simulink model "e5_Quadrotor_stable_nn_cex"  (R2020a)
settings: Solver=FixedStepAuto  StartTime=0.0  StopTime=options.T_train  FixedStep=options.dt  RelTol=1e-6
undefined symbols (not defined in the file or in its folder): options, Quad
libraries: neural x179, simulink x3
(part 5 of 10)

== system e5_Quadrotor_stable_nn_cex/NN/Layer 2/Delays 1 ==
  "p{2}" : Inport  PortDimensions=50
      mask Display: e = 0.06;c1 = [120 230 180]/255;c2 = ([120 230 180]+0)/(256+128);c3 = ([120 230 180]+128)/(256+128);patch([0 1 1 0],[0 0 1 1],c1);patch([0 1 1 1-e 1-e 0+e],[0 0 1 1-e 0+e 0+e],c2);patch([0 0 1 1-e 0+e 0+e],[0 1 1 1-e 1-e 0+e],c3);plot([0 1 1 0 0],[0 0 1 1 0]);
  mux : Mux  Inputs=1
      mask Display: e = 0.06;c1 = [120 150 230]/255;c2 = ([120 150 230]+0)/383;c3 = ([120 150 230]+128)/383;patch([0 1 1 0],[0 0 1 1],c1);patch([0 1 1 1-e 1-e 0+e],[0 0 1 1-e 0+e 0+e],c2);patch([0 0 1 1-e 0+e 0+e],[0 1 1 1-e 1-e 0+e],c3);plot([0 1 1 0 0],[0 0 1 1 0]);disp('Mux')
  "pd{2,1}" : Outport
      mask Display: e = 0.06;c1 = [120 230 180]/255;c2 = ([120 230 180]+0)/(256+128);c3 = ([120 230 180]+128)/(256+128);patch([0 1 1 0],[0 0 1 1],c1);patch([0 1 1 1-e 1-e 0+e],[0 0 1 1-e 0+e 0+e],c2);patch([0 0 1 1-e 0+e 0+e],[0 1 1 1-e 1-e 0+e],c3);plot([0 1 1 0 0],[0 0 1 1 0]);
  wires:
  "p{2}"/1 -> mux/1
  mux/1 -> "pd{2,1}"/1

== system e5_Quadrotor_stable_nn_cex/NN/Layer 2/LW{2,1} ==
  "ad{2,1}" : Inport  PortDimensions=50
      mask Display: e = 0.06;c1 = [120 230 180]/255;c2 = ([120 230 180]+0)/(256+128);c3 = ([120 230 180]+128)/(256+128);patch([0 1 1 0],[0 0 1 1],c1);patch([0 1 1 1-e 1-e 0+e],[0 0 1 1-e 0+e 0+e],c2);patch([0 0 1 1-e 0+e 0+e],[0 1 1 1-e 1-e 0+e],c3);plot([0 1 1 0 0],[0 0 1 1 0]);
  "IW{2,1}(1,:)'" : Constant  Value=[0.307987499556904686937031101479078643023967742919921875;-0.1426490927245896711550443569649360142648220062255859375;0.3186904457565054027412543291575275361537933349609375;0.07985545862075597856044595346247660927474498748779296875;0.1025200968211302521293504241839400492608547210693359375;0.0743281522622597778937603152371593751013278961181640625;0.0461591228672471876048888361765420995652675628662109375;-0.29902961209773104567233303896500729024410247802734375;0.55815593228456916730095827006152831017971038818359375;-0.408925703615676761071284772697254084050655364990234375;-0.260167952711846617308566464998875744640827178955078125;-0.5716920292723466356932249254896305501461029052734375;-0.54571618393627108201116016061860136687755584716796875;-0.51085748334703839912407374868053011596202850341796875;0.462878941862422121911180283859721384942531585693359375;-0.252711373418133600221580081779393367469310760498046875;-0.42051854980288794205733893249998800456523895263671875;-0.2349564558800354141521182782526011578738689422607421875;-1.189484931950835377989506014273501932621002197265625;-0.3623281949587722206018725046305917203426361083984375;-1.563420489812857194777961922227405011653900146484375;-3.137315439508801429013828965253196656703948974609375;-0.02477890272713605124277336244631442241370677947998046875;0.055931837035923755163668857903758180327713489532470703125;1.5119274342831385826713130882126279175281524658203125;0.02797521714572741291515711736792582087218761444091796875;-0.2404878929803591358638215069731813855469226837158203125;2.894986378812223648537838016636669635772705078125;-2.376549890337282366914450904005207121372222900390625;0.392571078539173445864918221559491939842700958251953125;-0.11848579033439331220645129860713495872914791107177734375;-0.0170814329101416084721876131879980675876140594482421875;0.460850686801575537554498396275448612868785858154296875;-0.489450805350698459061931089308927766978740692138671875;1.448186729572959574596779930288903415203094482421875;0.90875106841217456743464708779356442391872406005859375;-0.11121066569125272194273890136173577047884464263916015625;-0.25716503441926452655508228417602367699146270751953125;-0.25228751046263864221685935262939892709255218505859375;-0.6565814212843112951389912268496118485927581787109375;0.730122842221971435350269530317746102809906005859375;-0.199454001687219661942407356036710552871227264404296875;0.36830619325244651207640345091931521892547607421875;-0.0253273449438266747002490575368938152678310871124267578125;0.58711428567857648630479161511175334453582763671875;-0.215458016498742688238365872166468761861324310302734375;0.57286040908468749410786813314189203083515167236328125;0.08872721465650824923532269394854665733873844146728515625;-0.126593723768970323195759419832029379904270172119140625;0.22726020862804630073839007309288717806339263916015625]
      mask Display: e = 0.06;c1 = [120 150 230]/255;c2 = ([120 150 230]+0)/383;c3 = ([120 150 230]+128)/383;patch([0 1 1 0],[0 0 1 1],c1);patch([0 1 1 1-e 1-e 0+e],[0 0 1 1-e 0+e 0+e],c2);patch([0 0 1 1-e 0+e 0+e],[0 1 1 1-e 1-e 0+e],c3);plot([0 1 1 0 0],[0 0 1 1 0]);disp('weights');
  "IW{2,1}(2,:)'" : Constant  Value=[-0.0747046850734229550550224985272507183253765106201171875;-0.062078910778490196953338653429455007426440715789794921875;-0.349447843589094697680508261328213848173618316650390625;0.13768626788985949271904019042267464101314544677734375;-0.00395786183621708344271272750347634428180754184722900390625;0.7083343767292993309325765949324704706668853759765625;0.4094463717699305949082599909161217510700225830078125;0.384943570941259027851089058458455838263034820556640625;0.2197894162525433348065462269005365669727325439453125;0.7117280508388563742272481249528937041759490966796875;-0.08328667464921846175229802611283957958221435546875;-0.51818444979461097954498427498037926852703094482421875;-0.0275318422735666527845221907000450300984084606170654296875;0.29109923794683656428361473444965668022632598876953125;0.35412903248418092783111887911218218505382537841796875;-0.267495448479441011446766651715734042227268218994140625;-0.61680863179752598579597133721108548343181610107421875;-0.063450246473022275939257497157086618244647979736328125;-0.37149941577737022324612325974158011376857757568359375;-0.2092502686562911495826710961409844458103179931640625;2.465734858085689484852309760753996670246124267578125;0.369141219899319528163772474727011285722255706787109375;0.07768271801814781440942425660978187806904315948486328125;0.08483747433343634403168920243842876516282558441162109375;-0.975735029296679545751658224617131054401397705078125;-0.1626146551020306585400021504028700292110443115234375;-0.265746564266609419657783064394607208669185638427734375;-2.473889784492789178926841486827470362186431884765625;-0.48728113785874171970391444119741208851337432861328125;0.177112793967637294212380538738216273486614227294921875;-0.2080370875396501395560022729114280082285404205322265625;-0.1069716997996704999085437748362892307341098785400390625;-0.40792196685078219164921620176755823194980621337890625;0.298575833759055553340289179686806164681911468505859375;-2.58914085782789271661386010237038135528564453125;-0.61505863630175472422934035421349108219146728515625;-0.313864718056906522036797468899749219417572021484375;-0.0851413920473089447238379534610430710017681121826171875;0.811660732668295192837604190572164952754974365234375;-0.011529022588921238046122397236104006879031658172607421875;0.2183765773654703090667084097731276415288448333740234375;0.2778436976735807473204431516933254897594451904296875;0.288516534415056369322627460860530845820903778076171875;-0.27466903328420499974527047015726566314697265625;0.446781171973608337566474801860749721527099609375;-0.301165163687790116142650731489993631839752197265625;0.98090658917839246289105403775465674698352813720703125;-0.193508103633629857664999462940613739192485809326171875;-0.50386267112586213823277603296446613967418670654296875;-0.143467614263104226157707898892113007605075836181640625]
      mask Display: e = 0.06;c1 = [120 150 230]/255;c2 = ([120 150 230]+0)/383;c3 = ([120 150 230]+128)/383;patch([0 1 1 0],[0 0 1 1],c1);patch([0 1 1 1-e 1-e 0+e],[0 0 1 1-e 0+e 0+e],c2);patch([0 0 1 1-e 0+e 0+e],[0 1 1 1-e 1-e 0+e],c3);plot([0 1 1 0 0],[0 0 1 1 0]);disp('weights');
  Mux : Mux  Inputs=2
      mask Display: e = 0.06;c1 = [120 150 230]/255;c2 = ([120 150 230]+0)/383;c3 = ([120 150 230]+128)/383;patch([0 1 1 0],[0 0 1 1],c1);patch([0 1 1 1-e 1-e 0+e],[0 0 1 1-e 0+e 0+e],c2);patch([0 0 1 1-e 0+e 0+e],[0 1 1 1-e 1-e 0+e],c3);plot([0 1 1 0 0],[0 0 1 1 0]);disp('Mux');
  dotprod1 : neural/Weight Functions/dotprod
  dotprod2 : neural/Weight Functions/dotprod
  "lz{2,1}" : Outport
      mask Display: e = 0.06;c1 = [120 230 180]/255;c2 = ([120 230 180]+0)/(256+128);c3 = ([120 230 180]+128)/(256+128);patch([0 1 1 0],[0 0 1 1],c1);patch([0 1 1 1-e 1-e 0+e],[0 0 1 1-e 0+e 0+e],c2);patch([0 0 1 1-e 0+e 0+e],[0 1 1 1-e 1-e 0+e],c3);plot([0 1 1 0 0],[0 0 1 1 0]);
  wires:
  "IW{2,1}(1,:)'"/1 -> dotprod1/1
  "ad{2,1}"/1 -> dotprod1/2, dotprod2/2
  dotprod1/1 -> Mux/1
  "IW{2,1}(2,:)'"/1 -> dotprod2/1
  dotprod2/1 -> Mux/2
  Mux/1 -> "lz{2,1}"/1

== system e5_Quadrotor_stable_nn_cex/NN_cex_1/Layer 1/Delays 1 ==
  "p{1}" : Inport  PortDimensions=15
      mask Display: e = 0.06;c1 = [120 230 180]/255;c2 = ([120 230 180]+0)/(256+128);c3 = ([120 230 180]+128)/(256+128);patch([0 1 1 0],[0 0 1 1],c1);patch([0 1 1 1-e 1-e 0+e],[0 0 1 1-e 0+e 0+e],c2);patch([0 0 1 1-e 0+e 0+e],[0 1 1 1-e 1-e 0+e],c3);plot([0 1 1 0 0],[0 0 1 1 0]);
  mux : Mux  Inputs=1
      mask Display: e = 0.06;c1 = [120 150 230]/255;c2 = ([120 150 230]+0)/383;c3 = ([120 150 230]+128)/383;patch([0 1 1 0],[0 0 1 1],c1);patch([0 1 1 1-e 1-e 0+e],[0 0 1 1-e 0+e 0+e],c2);patch([0 0 1 1-e 0+e 0+e],[0 1 1 1-e 1-e 0+e],c3);plot([0 1 1 0 0],[0 0 1 1 0]);disp('Mux')
  "pd{1,1}" : Outport
      mask Display: e = 0.06;c1 = [120 230 180]/255;c2 = ([120 230 180]+0)/(256+128);c3 = ([120 230 180]+128)/(256+128);patch([0 1 1 0],[0 0 1 1],c1);patch([0 1 1 1-e 1-e 0+e],[0 0 1 1-e 0+e 0+e],c2);patch([0 0 1 1-e 0+e 0+e],[0 1 1 1-e 1-e 0+e],c3);plot([0 1 1 0 0],[0 0 1 1 0]);
  wires:
  "p{1}"/1 -> mux/1
  mux/1 -> "pd{1,1}"/1
